simulink model "Controlled_simulink_model"  (R2021a)
settings: Solver=VariableStepAuto  StartTime=0  StopTime=150  FixedStep=0.001  MaxStep=1e-4  MinStep=1e-5  RelTol=1e-5
values from neighbouring files (symbols this model uses):
  Accel_bias = 0    [Controlled_model.m]
  Amps = C/1000    (= 0.7)    [Controlled_model.m]
  Ax = 0.0    (= 0)    [Controlled_model.m]
  Ay = 0.0    (= 0)    [Controlled_model.m]
  b = 1.144e-08    [Controlled_model.m]
  b_m = 2.415e-6    (= 2.415e-06)    [Controlled_model.m]
  CD = 60    [Controlled_model.m]
  d = 9.94e-10    [Controlled_model.m]
  g = 9.81    [Controlled_model.m]
  Gyro_bias = 0    [Controlled_model.m]
  Ixx = 7.5*10^(-3)    (= 0.0075)    [Controlled_model.m]
  Iyy = 7.5*10^(-3)    (= 0.0075)    [Controlled_model.m]
  Izz = 1.3*10^(-2)    (= 0.013)    [Controlled_model.m]
  Jr = 6.5*10^(-7)    (= 6.5e-07)    [Controlled_model.m]
  Kemf = 0.00255    [Controlled_model.m]
  Kt = Kemf    (= 0.00255)    [Controlled_model.m]
  l = 0.23    [Controlled_model.m]
  L = 0.001*R    (= 0.000117)    [Controlled_model.m]
  m = weight/g    (= 0.0289500509684)    [Controlled_model.m]
  PD = 120    [Controlled_model.m]
  R = 0.117    [Controlled_model.m]
undefined symbols (not defined in the file or in its folder): Ion, Lithium, sigbuilder_block
libraries: simulink x9, visionstatistics x1, spsControlledCurrentSourceLib x1, spsBatteryLib x1, spspowerguiLib x1
settings Model: Creator=Nicky  LastModifiedBy=YeBobo
settings SolverCC: MaxConsecutiveZCs=500  MaxConsecutiveMinStep=100  ZeroCrossAlgorithm=Adaptive  AlgebraicLoopSolver=LineSearch  AutoInsertRateTranBlk=on
settings DataIOCC: ReturnWorkspaceOutputs=off
settings DebuggingCC: MaxConsecutiveZCsMsg=none  SFMachineParentedDataDiag=warning  ArithmeticOperatorsInVariantConditions=warning
settings SFSimCC: SimUseLocalCustomCode=off  CustomCodeUndefinedFunction=UseInterfaceOnly
settings RTWCC: RTWUseLocalCustomCode=off
settings CodeAppCC: StateflowObjectComments=on
settings SimscapeCC: SimscapeNormalizeSystem=off

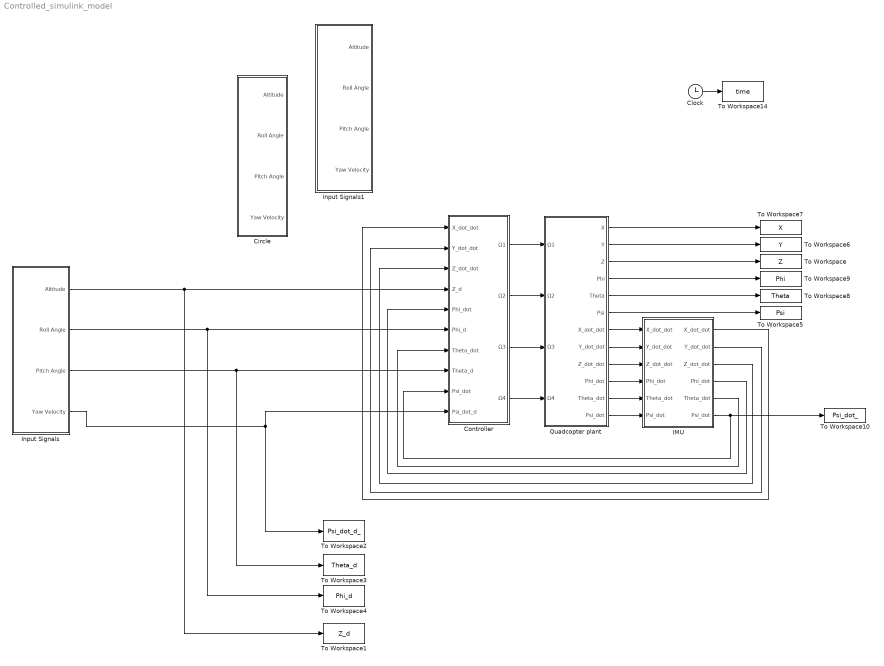
== system Controlled_simulink_model ==
  Circle : Subsystem  Tag=STV Subsys  LoadFcn=sigbuilder_block('load');  StartFcn=sigbuilder_block('start');  StopFcn=sigbuilder_block('stop');  ClipboardFcn=sigbuilder_block('clipboard');  mask(Sigbuilder block){tuvar=[0:10]}
      mask help: Simulink:masks:SigbuilderBlock_MD
      mask init:
      | if ~strcmp(get_param(bdroot(gcbh),'SimulationStatus'),'stopped') tuvar = sigbuilder_block('maskInit'); end
      settings: CopyFcn=sigbuilder_block('copy');  DeleteFcn=sigbuilder_block('delete');  ModelCloseFcn=sigbuilder_block('modelClose');  PreSaveFcn=sigbuilder_block('preSave');  PauseFcn=sigbuilder_block('pause');  ContinueFcn=sigbuilder_block('continue');  NameChangeFcn=sigbuilder_block('namechange');  OpenFcn=sigbuilder_block('open',[173.25 183.75 1012.5 456 ]);  CloseFcn=sigbuilder_block('close');
      mask Display: plot(0, 0, 100, 100,[2, 2, 32, 32, 2], [68, 8, 8, 68, 68],[32, 2], [38, 38], [32, 19, 2],[53, 60, 44], [32, 17, 17, 2],[16, 16, 31, 31]);txt = getActiveGroup(gcbh);text(2, 100, txt,'verticalAlignment', 'top');
  Clock : Clock
  Controller : Subsystem
  IMU : Subsystem
  Input Signals : Subsystem  Tag=STV Subsys  LoadFcn=sigbuilder_block('load');  StartFcn=sigbuilder_block('start');  StopFcn=sigbuilder_block('stop');  ClipboardFcn=sigbuilder_block('clipboard');  mask(Sigbuilder block){tuvar=[0:10]}
      mask help: Simulink:masks:SigbuilderBlock_MD
      mask init:
      | if ~strcmp(get_param(bdroot(gcbh),'SimulationStatus'),'stopped') tuvar = sigbuilder_block('maskInit'); end
      settings: CopyFcn=sigbuilder_block('copy');  DeleteFcn=sigbuilder_block('delete');  ModelCloseFcn=sigbuilder_block('modelClose');  PreSaveFcn=sigbuilder_block('preSave');  PauseFcn=sigbuilder_block('pause');  ContinueFcn=sigbuilder_block('continue');  NameChangeFcn=sigbuilder_block('namechange');  OpenFcn=sigbuilder_block('open',[133.8 179.4 1012.8 407.4 ]);  CloseFcn=sigbuilder_block('close');
      mask Display: plot(0, 0, 100, 100,[2, 2, 32, 32, 2], [68, 8, 8, 68, 68],[32, 2], [38, 38], [32, 19, 2],[53, 60, 44], [32, 17, 17, 2],[16, 16, 31, 31]);txt = getActiveGroup(gcbh);text(2, 100, txt,'verticalAlignment', 'top');
  Input Signals1 : Subsystem  Tag=STV Subsys  LoadFcn=sigbuilder_block('load');  StartFcn=sigbuilder_block('start');  StopFcn=sigbuilder_block('stop');  ClipboardFcn=sigbuilder_block('clipboard');  mask(Sigbuilder block){tuvar=[0:10]}
      mask help: Simulink:masks:SigbuilderBlock_MD
      mask init:
      | if ~strcmp(get_param(bdroot(gcbh),'SimulationStatus'),'stopped') tuvar = sigbuilder_block('maskInit'); end
      settings: CopyFcn=sigbuilder_block('copy');  DeleteFcn=sigbuilder_block('delete');  ModelCloseFcn=sigbuilder_block('modelClose');  PreSaveFcn=sigbuilder_block('preSave');  PauseFcn=sigbuilder_block('pause');  ContinueFcn=sigbuilder_block('continue');  NameChangeFcn=sigbuilder_block('namechange');  OpenFcn=sigbuilder_block('open',[369 232.5 1012.5 445.5 ]);  CloseFcn=sigbuilder_block('close');
      mask Display: plot(0, 0, 100, 100,[2, 2, 32, 32, 2], [68, 8, 8, 68, 68],[32, 2], [38, 38], [32, 19, 2],[53, 60, 44], [32, 17, 17, 2],[16, 16, 31, 31]);txt = getActiveGroup(gcbh);text(2, 100, txt,'verticalAlignment', 'top');
  Quadcopter plant : Subsystem
  To Workspace : ToWorkspace  VariableName=Z  SampleTime=0.001
      settings: Save2DSignal=2-D array (concatenate along first dimension)
  To Workspace1 : ToWorkspace  VariableName=Z_d  SampleTime=0.001
      settings: Save2DSignal=2-D array (concatenate along first dimension)
  To Workspace10 : ToWorkspace  VariableName=Psi_dot_  SampleTime=0.001
      settings: Save2DSignal=2-D array (concatenate along first dimension)
  To Workspace14 : ToWorkspace  VariableName=time  SampleTime=0.001
      settings: Save2DSignal=2-D array (concatenate along first dimension)
  To Workspace2 : ToWorkspace  VariableName=Psi_dot_d_  SampleTime=0.001
      settings: Save2DSignal=2-D array (concatenate along first dimension)
  To Workspace3 : ToWorkspace  VariableName=Theta_d  SampleTime=0.001
      settings: Save2DSignal=2-D array (concatenate along first dimension)
  To Workspace4 : ToWorkspace  VariableName=Phi_d  SampleTime=0.001
      settings: Save2DSignal=2-D array (concatenate along first dimension)
  To Workspace5 : ToWorkspace  VariableName=Psi  SampleTime=0.001
      settings: Save2DSignal=2-D array (concatenate along first dimension)
  To Workspace6 : ToWorkspace  VariableName=Y  SampleTime=0.001
      settings: Save2DSignal=2-D array (concatenate along first dimension)
  To Workspace7 : ToWorkspace  VariableName=X  SampleTime=0.001
      settings: Save2DSignal=2-D array (concatenate along first dimension)
  To Workspace8 : ToWorkspace  VariableName=Theta  SampleTime=0.001
      settings: Save2DSignal=2-D array (concatenate along first dimension)
  To Workspace9 : ToWorkspace  VariableName=Phi  SampleTime=0.001
      settings: Save2DSignal=2-D array (concatenate along first dimension)
  wires:
  Clock/1 -> To Workspace14/1
  Controller/1(Ω1) -> Quadcopter plant/1(Ω1)
  Controller/2(Ω2) -> Quadcopter plant/2(Ω2)
  Controller/3(Ω3) -> Quadcopter plant/3(Ω3)
  Controller/4(Ω4) -> Quadcopter plant/4(Ω4)
  IMU/6("Psi_dot ") -> Controller/9(Psi_dot), To Workspace10/1
  IMU/5("Theta_dot ") -> Controller/7(Theta_dot)
  IMU/3("Z_dot_dot ") -> Controller/3(Z_dot_dot)
  Quadcopter plant/1(X) -> To Workspace7/1
  Quadcopter plant/2(Y) -> To Workspace6/1
  Quadcopter plant/3(Z) -> To Workspace/1
  Quadcopter plant/7(X_dot_dot) -> IMU/1(X_dot_dot)
  Quadcopter plant/8("Y_dot_dot ") -> IMU/2(Y_dot_dot)
  Quadcopter plant/9(Z_dot_dot) -> IMU/3(Z_dot_dot)
  Quadcopter plant/11(Theta_dot) -> IMU/5(Theta_dot)
  Quadcopter plant/10(Phi_dot) -> IMU/4(Phi_dot)
  Quadcopter plant/12(Psi_dot) -> IMU/6(Psi_dot)
  Quadcopter plant/5(Theta) -> To Workspace8/1
  Quadcopter plant/6(Psi) -> To Workspace5/1
  IMU/2("Y_dot_dot ") -> Controller/2(Y_dot_dot)
  Input Signals/4(Yaw Velocity) -> Controller/10(Psi_dot_d), To Workspace2/1
  IMU/4("Phi_dot ") -> Controller/5(Phi_dot)
  Quadcopter plant/4(Phi) -> To Workspace9/1
  Input Signals/1(Altitude) -> To Workspace1/1, Controller/4(Z_d)
  Input Signals/2(Roll Angle) -> To Workspace4/1, Controller/6(Phi_d)
  Input Signals/3(Pitch Angle) -> To Workspace3/1, Controller/8(Theta_d)
  IMU/1("X_dot_dot ") -> Controller/1(X_dot_dot)

== system Controlled_simulink_model/Circle ==
  Demux : Demux  Tag=STV Demux
      settings: DisplayOption=none
  FromWs : FromWorkspace  Tag=STV FromWs  VariableName=tuvar
      SigBuilderData=|
      | common.afterFinalStr = 'Extrapolate'
      | common.sampleTime = 0
      | dataSet.timeRange = [0 150]
      | dataSet.name = 'Group 1'
      | sbobj.Groups.Name = 'Group 1'
      | sbobj.Groups.Signals(1).Name = 'Altitude'
      | sbobj.Groups.Signals(1).XData = [0 1 150]
      | sbobj.Groups.Signals(1).YData = [0 1 5]
      | sbobj.Groups.Signals(2).Name = 'Roll Angle'
      | sbobj.Groups.Signals(2).XData = [0 13 14 18 20 29 31 40 42 51 53 62 64 73 75 84 86 95 97 106 108 117 119 128 130 139 141 150]
      | sbobj.Groups.Signals(2).YData = [0 0 -0.1 -0.1 0.1 0.1 -0.1 -0.1 0.1 0.1 -0.1 -0.1 0.1 0.1 -0.1 -0.1 0.1 0.1 -0.1 -0.1 0.1 0.1 -0.1 -0.1 0.1 0.1 -0.1 -0.1]
      | sbobj.Groups.Signals(3).Name = 'Pitch Angle'
      | sbobj.Groups.Signals(3).XData = [0 7 8 12 14 23 25 34 36 45 47 56 58 67 69 78 80 89 91 100 102 111 113 122 124 133 135 144 146 150]
      | sbobj.Groups.Signals(3).YData = [0 0 -0.1 -0.1 0.1 0.1 -0.1 -0.1 0.1 0.1 -0.1 -0.1 0.1 0.1 -0.1 -0.1 0.1 0.1 -0.1 -0.1 0.1 0.1 -0.1 -0.1 0.1 0.1 -0.1 -0.1 0 0]
      | sbobj.Groups.Signals(4).Name = 'Yaw Velocity'
      | sbobj.Groups.Signals(4).XData = [0 150]
      | sbobj.Groups.Signals(4).YData = [0 0]
      | sbobj.Groups.TimeRange = [0 150]
  Altitude : Outport  Tag=STV Outport  VectorParamsAs1DForOutWhenUnconnected=off
  Roll Angle : Outport  Tag=STV Outport  Port=2  VectorParamsAs1DForOutWhenUnconnected=off
  Pitch Angle : Outport  Tag=STV Outport  Port=3  VectorParamsAs1DForOutWhenUnconnected=off
  Yaw Velocity : Outport  Tag=STV Outport  Port=4  VectorParamsAs1DForOutWhenUnconnected=off
  wires:
  FromWs/1 -> Demux/1
  Demux/1 -> Altitude/1
  Demux/2 -> Roll Angle/1
  Demux/3 -> Pitch Angle/1
  Demux/4 -> Yaw Velocity/1

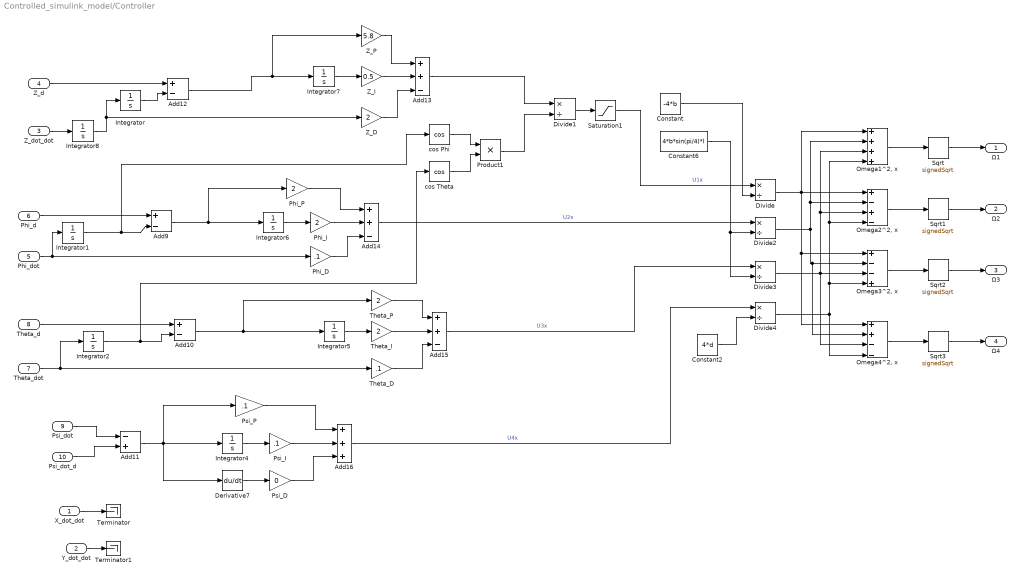
== system Controlled_simulink_model/Controller ==
  X_dot_dot : Inport
  Y_dot_dot : Inport  Port=2
  Z_dot_dot : Inport  Port=3
  Z_d : Inport  Port=4
  Phi_dot : Inport  Port=5
  Phi_d : Inport  Port=6
  Theta_dot : Inport  Port=7
  Theta_d : Inport  Port=8
  Psi_dot : Inport  Port=9
  Psi_dot_d : Inport  Port=10
  Add10 : Sum  Inputs=+-
  Add11 : Sum  Inputs=-+
  Add12 : Sum  Inputs=+-
  Add13 : Sum  Inputs=++-
  Add14 : Sum  Inputs=++-
  Add15 : Sum  Inputs=++-
  Add16 : Sum  Inputs=+++
  Add9 : Sum  Inputs=+-
  Constant : Constant  Value=-4*b
  Constant2 : Constant  Value=4*d
  Constant6 : Constant  Value=4*b*sin(pi/4)*l
  Derivative7 : Derivative
  Divide{,1..4} (5 alike) : Product  Inputs=*/
  Integrator : Integrator  LimitOutput=on  UpperSaturationLimit=0
  Integrator1 : Integrator  WrapState=on
  Integrator2 : Integrator  WrapState=on
  Integrator{4..8} (5 alike) : Integrator
  "Omega1^2, x" : Sum  Inputs=++++
  "Omega2^2, x" : Sum  Inputs=+-+-
  "Omega3^2, x" : Sum  Inputs=+--+
  "Omega4^2, x" : Sum  Inputs=++--
  Phi_D : Gain  Gain=.1
  Phi_I : Gain  Gain=2
  Phi_P : Gain  Gain=2
  Product1 : Product  RndMeth=Zero
  Psi_D : Gain  Gain=0
  Psi_I : Gain  Gain=.1
  Psi_P : Gain  Gain=.1
  Saturation1 : Saturate  UpperLimit=0  LowerLimit=-inf
  Sqrt{,1..3} (4 alike) : Sqrt  Operator=signedSqrt  SaturateOnIntegerOverflow=on
  Terminator : Terminator
  Terminator1 : Terminator
  Theta_D : Gain  Gain=.1
  Theta_I : Gain  Gain=2
  Theta_P : Gain  Gain=2
  Z_D : Gain  Gain=2
  "Z_I " : Gain  Gain=0.5
  Z_P : Gain  Gain=5.8
  cos Phi : Trigonometry  Operator=cos
  cos Theta : Trigonometry  Operator=cos
  Ω1 : Outport  VectorParamsAs1DForOutWhenUnconnected=off
  Ω2 : Outport  Port=2  VectorParamsAs1DForOutWhenUnconnected=off
  Ω3 : Outport  Port=3  VectorParamsAs1DForOutWhenUnconnected=off
  Ω4 : Outport  Port=4  VectorParamsAs1DForOutWhenUnconnected=off
  wires:
  Z_D/1 -> Add13/3
  Theta_I/1 -> Add15/2
  Add12/1 -> Z_P/1, Integrator7/1
  Z_dot_dot/1 -> Integrator8/1
  Add11/1 -> Derivative7/1, Integrator4/1, Psi_P/1
  "Z_I "/1 -> Add13/2
  Theta_P/1 -> Add15/1
  Integrator4/1 -> Psi_I/1
  Integrator7/1 -> "Z_I "/1
  Add9/1 -> Integrator6/1, Phi_P/1
  Derivative7/1 -> Psi_D/1
  Psi_D/1 -> Add16/3
  Psi_I/1 -> Add16/2
  Integrator6/1 -> Phi_I/1
  cos Theta/1 -> Product1/2
  Add13/1 -> Divide1/1
  Phi_dot/1 -> Phi_D/1, Integrator1/1
  Phi_D/1 -> Add14/3
  cos Phi/1 -> Product1/1
  Divide1/1 -> Saturation1/1
  Theta_D/1 -> Add15/3
  Integrator5/1 -> Theta_I/1
  Add10/1 -> Theta_P/1, Integrator5/1
  Product1/1 -> Divide1/2
  Phi_I/1 -> Add14/2
  Theta_dot/1 -> Integrator2/1, Theta_D/1
  Phi_P/1 -> Add14/1
  Psi_P/1 -> Add16/1
  Z_P/1 -> Add13/1
  Constant6/1 -> Divide3/2, Divide2/2
  Add14/1 -> Divide2/1  "U2x"
  Add15/1 -> Divide3/1  "U3x"
  Saturation1/1 -> Divide/1  "U1x"
  Constant/1 -> Divide/2
  Constant2/1 -> Divide4/2
  Add16/1 -> Divide4/1  "U4x"
  Sqrt/1 -> Ω1/1
  Sqrt1/1 -> Ω2/1
  Sqrt2/1 -> Ω3/1
  Sqrt3/1 -> Ω4/1
  Divide4/1 -> "Omega3^2, x"/4, "Omega2^2, x"/4, "Omega1^2, x"/4, "Omega4^2, x"/4
  Divide2/1 -> "Omega4^2, x"/2, "Omega3^2, x"/2, "Omega2^2, x"/2, "Omega1^2, x"/2
  Divide3/1 -> "Omega4^2, x"/3, "Omega3^2, x"/3, "Omega2^2, x"/3, "Omega1^2, x"/3
  Divide/1 -> "Omega4^2, x"/1, "Omega3^2, x"/1, "Omega2^2, x"/1, "Omega1^2, x"/1
  "Omega1^2, x"/1 -> Sqrt/1
  "Omega2^2, x"/1 -> Sqrt1/1
  "Omega3^2, x"/1 -> Sqrt2/1
  "Omega4^2, x"/1 -> Sqrt3/1
  Z_d/1 -> Add12/1
  Phi_d/1 -> Add9/1
  Integrator1/1 -> cos Phi/1, Add9/2
  Integrator2/1 -> cos Theta/1, Add10/2
  Theta_d/1 -> Add10/1
  Psi_dot/1 -> Add11/1
  Psi_dot_d/1 -> Add11/2
  Integrator/1 -> Add12/2
  Integrator8/1 -> Z_D/1, Integrator/1
  X_dot_dot/1 -> Terminator/1
  Y_dot_dot/1 -> Terminator1/1

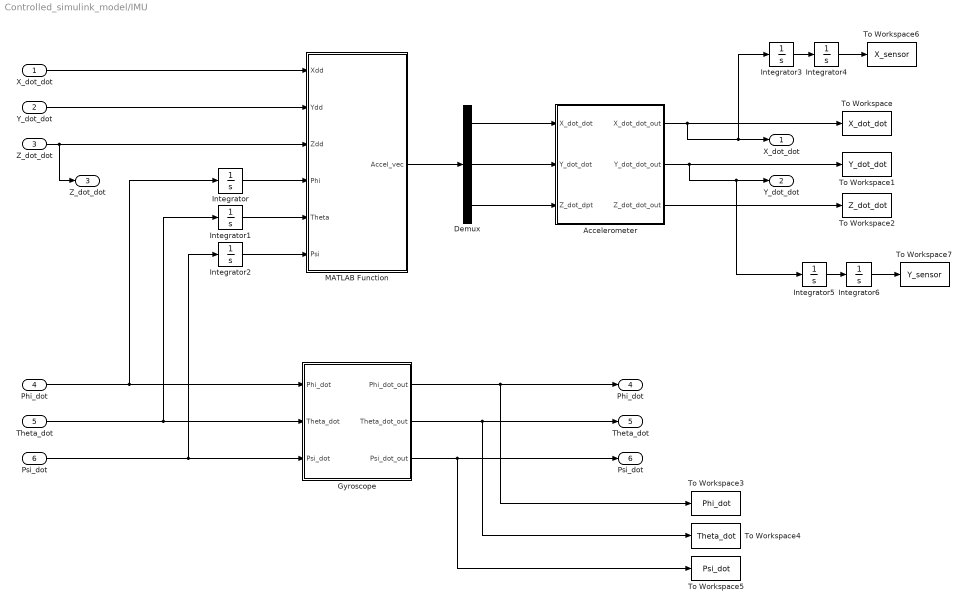
== system Controlled_simulink_model/IMU ==
  X_dot_dot : Inport
  Y_dot_dot : Inport  Port=2
  Z_dot_dot : Inport  Port=3
  Phi_dot : Inport  Port=4
  Theta_dot : Inport  Port=5
  Psi_dot : Inport  Port=6
  Accelerometer : Subsystem
  Demux : Demux  Outputs=3
  Gyroscope : Subsystem
  Integrator : Integrator  WrapState=on
  Integrator1 : Integrator  WrapState=on
  Integrator{2..6} (5 alike) : Integrator
  MATLAB Function : MATLAB Function  TreatAsAtomicUnit=on
  To Workspace : ToWorkspace  VariableName=X_dot_dot  SampleTime=0.001
      settings: Save2DSignal=2-D array (concatenate along first dimension)
  To Workspace1 : ToWorkspace  VariableName=Y_dot_dot  SampleTime=0.001
      settings: Save2DSignal=2-D array (concatenate along first dimension)
  To Workspace2 : ToWorkspace  VariableName=Z_dot_dot  SampleTime=0.001
      settings: Save2DSignal=2-D array (concatenate along first dimension)
  To Workspace3 : ToWorkspace  VariableName=Phi_dot  SampleTime=0.001
      settings: Save2DSignal=2-D array (concatenate along first dimension)
  To Workspace4 : ToWorkspace  VariableName=Theta_dot  SampleTime=0.001
      settings: Save2DSignal=2-D array (concatenate along first dimension)
  To Workspace5 : ToWorkspace  VariableName=Psi_dot  SampleTime=0.001
      settings: Save2DSignal=2-D array (concatenate along first dimension)
  To Workspace6 : ToWorkspace  VariableName=X_sensor  SampleTime=0.001
      settings: Save2DSignal=2-D array (concatenate along first dimension)
  To Workspace7 : ToWorkspace  VariableName=Y_sensor  SampleTime=0.001
      settings: Save2DSignal=2-D array (concatenate along first dimension)
  "X_dot_dot " : Outport  VectorParamsAs1DForOutWhenUnconnected=off
  "Y_dot_dot " : Outport  Port=2  VectorParamsAs1DForOutWhenUnconnected=off
  "Z_dot_dot " : Outport  Port=3  VectorParamsAs1DForOutWhenUnconnected=off
  "Phi_dot " : Outport  Port=4  VectorParamsAs1DForOutWhenUnconnected=off
  "Theta_dot " : Outport  Port=5  VectorParamsAs1DForOutWhenUnconnected=off
  "Psi_dot " : Outport  Port=6  VectorParamsAs1DForOutWhenUnconnected=off
  wires:
  Phi_dot/1 -> Integrator/1, Gyroscope/1(Phi_dot)
  Theta_dot/1 -> Integrator1/1, Gyroscope/2(Theta_dot)
  Psi_dot/1 -> Integrator2/1, Gyroscope/3(Psi_dot)
  Gyroscope/2(Theta_dot_out) -> "Theta_dot "/1, To Workspace4/1
  Gyroscope/1(Phi_dot_out) -> "Phi_dot "/1, To Workspace3/1
  Accelerometer/1(X_dot_dot_out) -> To Workspace/1, Integrator3/1, "X_dot_dot "/1
  Accelerometer/3(Z_dot_dot_out) -> To Workspace2/1
  Gyroscope/3(Psi_dot_out) -> "Psi_dot "/1, To Workspace5/1
  X_dot_dot/1 -> MATLAB Function/1(Xdd)
  Y_dot_dot/1 -> MATLAB Function/2(Ydd)
  Z_dot_dot/1 -> "Z_dot_dot "/1, MATLAB Function/3(Zdd)
  Integrator/1 -> MATLAB Function/4(Phi)
  Integrator2/1 -> MATLAB Function/6(Psi)
  Integrator1/1 -> MATLAB Function/5(Theta)
  MATLAB Function/1(Accel_vec) -> Demux/1
  Demux/2 -> Accelerometer/2("Y_dot_dot ")
  Demux/1 -> Accelerometer/1(X_dot_dot)
  Demux/3 -> Accelerometer/3("Z_dot_dpt ")
  Integrator3/1 -> Integrator4/1
  Integrator4/1 -> To Workspace6/1
  Integrator6/1 -> To Workspace7/1
  Accelerometer/2(Y_dot_dot_out) -> Integrator5/1, "Y_dot_dot "/1, To Workspace1/1
  Integrator5/1 -> Integrator6/1

== system Controlled_simulink_model/Input Signals ==
  Demux : Demux  Tag=STV Demux
      settings: DisplayOption=none
  FromWs : FromWorkspace  Tag=STV FromWs  VariableName=tuvar
      SigBuilderData=|
      | common.afterFinalStr = 'Extrapolate'
      | common.sampleTime = 0
      | dataSet.timeRange = [0 150]
      | dataSet.name = 'Group 1'
      | sbobj.Groups.Name = 'Group 1'
      | sbobj.Groups.Signals(1).Name = 'Altitude'
      | sbobj.Groups.Signals(1).XData = [0 60 60 150]
      | sbobj.Groups.Signals(1).YData = [-1 -1 -2 -2]
      | sbobj.Groups.Signals(2).Name = 'Roll Angle'
      | sbobj.Groups.Signals(2).XData = [0 2 3 5 6 8 9 11 12 30 31 33 34 36 37 39 40 75 76 78 79 81 82 84 85 103 104 106 107 109 110 112 113 150]
      | sbobj.Groups.Signals(2).YData = [0 0 0.2 0.2 0 0 -0.2 -0.2 0 0 -0.2 -0.2 0 0 0.2 0.2 0 0 0.2 0.2 0 0 -0.2 -0.2 0 0 -0.2 -0.2 0 0 0.2 0.2 0 0]
      | sbobj.Groups.Signals(3).Name = 'Pitch Angle'
      | sbobj.Groups.Signals(3).XData = [0 16 17 19 20 22 23 25 26 44 45 47 48 50 51 53 54 89 90 92 93 95 96 98 99 117 117 118 120 121 123 124 126 127 140.4 150]
      | sbobj.Groups.Signals(3).YData = [0 0 0.2 0.2 0 0 -0.2 -0.2 0 0 -0.2 -0.2 0 0 0.2 0.2 0 0 0.2 0.2 0 0 -0.2 -0.2 0 0 0.005 -0.2 -0.2 0 0 0.2 0.2 0 0 0]
      | sbobj.Groups.Signals(4).Name = 'Yaw Velocity'
      | sbobj.Groups.Signals(4).XData = [0 65 66 70 71 150]
      | sbobj.Groups.Signals(4).YData = [0 0 0.5 0.5 0 0]
      | sbobj.Groups.TimeRange = [0 150]
  Altitude : Outport  Tag=STV Outport  VectorParamsAs1DForOutWhenUnconnected=off
  Roll Angle : Outport  Tag=STV Outport  Port=2  VectorParamsAs1DForOutWhenUnconnected=off
  Pitch Angle : Outport  Tag=STV Outport  Port=3  VectorParamsAs1DForOutWhenUnconnected=off
  Yaw Velocity : Outport  Tag=STV Outport  Port=4  VectorParamsAs1DForOutWhenUnconnected=off
  wires:
  FromWs/1 -> Demux/1
  Demux/1 -> Altitude/1
  Demux/2 -> Roll Angle/1
  Demux/3 -> Pitch Angle/1
  Demux/4 -> Yaw Velocity/1

== system Controlled_simulink_model/Input Signals1 ==
  Demux : Demux  Tag=STV Demux
      settings: DisplayOption=none
  FromWs : FromWorkspace  Tag=STV FromWs  VariableName=tuvar
      SigBuilderData=|
      | common.afterFinalStr = 'Extrapolate'
      | common.sampleTime = 0
      | dataSet.timeRange = [0 150]
      | dataSet.name = 'Group 1'
      | sbobj.Groups.Name = 'Group 1'
      | sbobj.Groups.Signals(1).Name = 'Altitude'
      | sbobj.Groups.Signals(1).XData = [0 150]
      | sbobj.Groups.Signals(1).YData = [-1 -10]
      | sbobj.Groups.Signals(2).Name = 'Roll Angle'
      | sbobj.Groups.Signals(2).XData = [0 2 3 5 6 16 17 19 20 30 31 33 34 44 45 47 48 103 104 106 107 109 110 112 113 150]
      | sbobj.Groups.Signals(2).YData = [0 0 0.2 0.2 0 0 -0.2 -0.2 0 0 0.2 0.2 0 0 -0.2 -0.2 0 0 -0.2 -0.2 0 0 0.2 0.2 0 0]
      | sbobj.Groups.Signals(3).Name = 'Pitch Angle'
      | sbobj.Groups.Signals(3).XData = [0 140.4 150]
      | sbobj.Groups.Signals(3).YData = [0 0 0]
      | sbobj.Groups.Signals(4).Name = 'Yaw Velocity'
      | sbobj.Groups.Signals(4).XData = [0 65 66 70 71 150]
      | sbobj.Groups.Signals(4).YData = [0 0 0.5 0.5 0 0]
      | sbobj.Groups.TimeRange = [0 150]
  Altitude : Outport  Tag=STV Outport  VectorParamsAs1DForOutWhenUnconnected=off
  Roll Angle : Outport  Tag=STV Outport  Port=2  VectorParamsAs1DForOutWhenUnconnected=off
  Pitch Angle : Outport  Tag=STV Outport  Port=3  VectorParamsAs1DForOutWhenUnconnected=off
  Yaw Velocity : Outport  Tag=STV Outport  Port=4  VectorParamsAs1DForOutWhenUnconnected=off
  wires:
  FromWs/1 -> Demux/1
  Demux/1 -> Altitude/1
  Demux/2 -> Roll Angle/1
  Demux/3 -> Pitch Angle/1
  Demux/4 -> Yaw Velocity/1

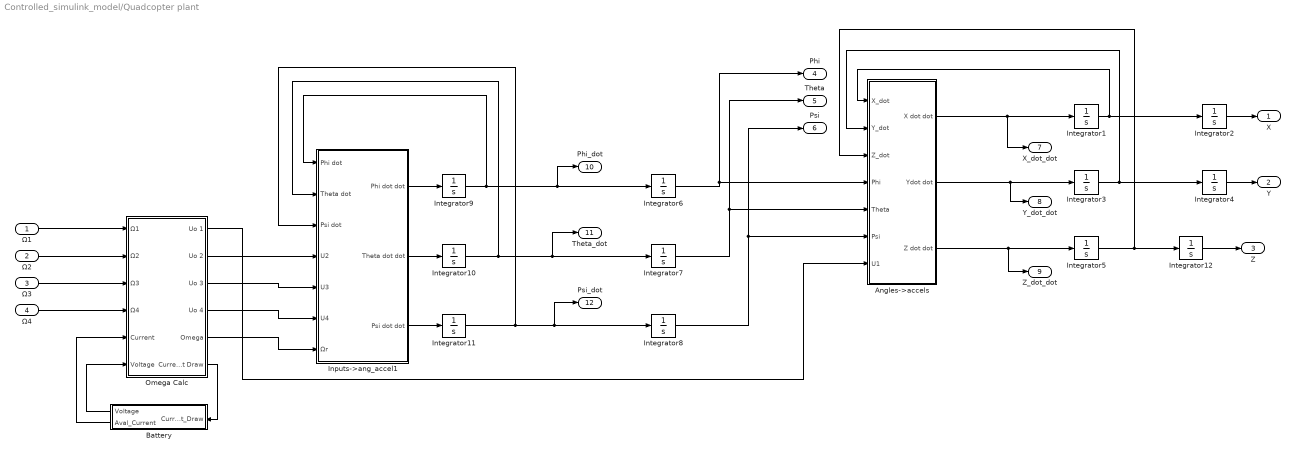
== system Controlled_simulink_model/Quadcopter plant ==
  Ω1 : Inport
  Ω2 : Inport  Port=2
  Ω3 : Inport  Port=3
  Ω4 : Inport  Port=4
  Angles->accels : Subsystem
  Battery : Subsystem
  Inputs->ang_accel1 : Subsystem
  Integrator{1..5,8..9} (7 alike) : Integrator
  Integrator10 : Integrator  IgnoreLimit=on
  Integrator11 : Integrator  UpperSaturationLimit=10000  LowerSaturationLimit=-10000
  Integrator12 : Integrator  LimitOutput=on  UpperSaturationLimit=0
  Integrator6 : Integrator  WrapState=on
  Integrator7 : Integrator  WrapState=on
  Omega Calc : Subsystem
  X : Outport  VectorParamsAs1DForOutWhenUnconnected=off
  Y : Outport  Port=2  VectorParamsAs1DForOutWhenUnconnected=off
  Z : Outport  Port=3  VectorParamsAs1DForOutWhenUnconnected=off
  Phi : Outport  Port=4  VectorParamsAs1DForOutWhenUnconnected=off
  Theta : Outport  Port=5  VectorParamsAs1DForOutWhenUnconnected=off
  Psi : Outport  Port=6  VectorParamsAs1DForOutWhenUnconnected=off
  X_dot_dot : Outport  Port=7  VectorParamsAs1DForOutWhenUnconnected=off
  "Y_dot_dot " : Outport  Port=8  VectorParamsAs1DForOutWhenUnconnected=off
  Z_dot_dot : Outport  Port=9  VectorParamsAs1DForOutWhenUnconnected=off
  Phi_dot : Outport  Port=10  VectorParamsAs1DForOutWhenUnconnected=off
  Theta_dot : Outport  Port=11  VectorParamsAs1DForOutWhenUnconnected=off
  Psi_dot : Outport  Port=12  VectorParamsAs1DForOutWhenUnconnected=off
  wires:
  Integrator7/1 -> Angles->accels/5(Theta), Theta/1
  Integrator6/1 -> Angles->accels/4(Phi), Phi/1
  Inputs->ang_accel1/2(Theta dot dot) -> Integrator10/1
  Inputs->ang_accel1/1(Phi dot dot) -> Integrator9/1
  Inputs->ang_accel1/3(Psi dot dot) -> Integrator11/1
  Omega Calc/5(Omega) -> Inputs->ang_accel1/7(Ωr)
  Omega Calc/4(Uo 4) -> Inputs->ang_accel1/6(U4)
  Omega Calc/3(Uo 3) -> Inputs->ang_accel1/5(U3)
  Omega Calc/2(Uo 2) -> Inputs->ang_accel1/4(U2)
  Omega Calc/1(Uo 1) -> Angles->accels/7(U1)
  Ω1/1 -> Omega Calc/1(Ω1)
  Ω2/1 -> Omega Calc/2(Ω2)
  Ω3/1 -> Omega Calc/3(Ω3)
  Ω4/1 -> Omega Calc/4(Ω4)
  Integrator9/1 -> Inputs->ang_accel1/1(Phi dot), Phi_dot/1, Integrator6/1
  Integrator11/1 -> Inputs->ang_accel1/3(Psi dot), Integrator8/1, Psi_dot/1
  Integrator10/1 -> Inputs->ang_accel1/2(Theta dot), Integrator7/1, Theta_dot/1
  Angles->accels/1(X dot dot) -> X_dot_dot/1, Integrator1/1
  Omega Calc/6(Current Draw) -> Battery/1(Current_Draw)
  Battery/1(Voltage) -> Omega Calc/6(Voltage)
  Battery/2(Aval_Current) -> Omega Calc/5(Current)
  Integrator1/1 -> Angles->accels/1(X_dot), Integrator2/1
  Integrator2/1 -> X/1
  Integrator3/1 -> Angles->accels/2(Y_dot), Integrator4/1
  Angles->accels/2(Ydot dot) -> "Y_dot_dot "/1, Integrator3/1
  Integrator4/1 -> Y/1
  Integrator5/1 -> Angles->accels/3(Z_dot), Integrator12/1
  Angles->accels/3(Z dot dot) -> Integrator5/1, Z_dot_dot/1
  Integrator12/1 -> Z/1
  Integrator8/1 -> Angles->accels/6(Psi), Psi/1

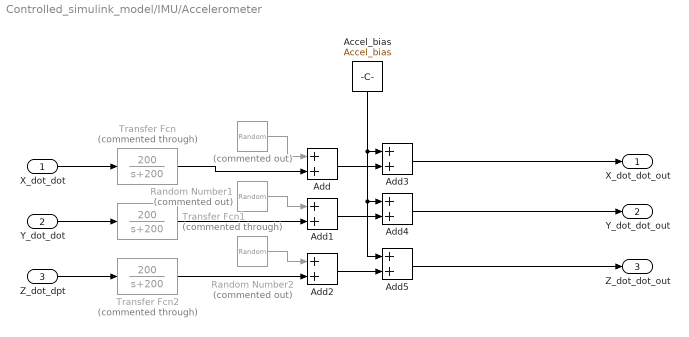
== system Controlled_simulink_model/IMU/Accelerometer ==
  X_dot_dot : Inport
  "Y_dot_dot " : Inport  Port=2
  "Z_dot_dpt " : Inport  Port=3
  " " : RandomNumber  Commented=on  Variance=0.0001  Seed=1  SampleTime=0.001
  Accel_bias : Constant  Value=Accel_bias
  Add{,1..5} (6 alike) : Sum
  Random Number1 : RandomNumber  Commented=on  Variance=0.0001  Seed=2  SampleTime=0.001
  Random Number2 : RandomNumber  Commented=on  Mean=0.000  Variance=0.0001  Seed=3  SampleTime=0.001
  Transfer Fcn : TransferFcn  Commented=through  Numerator=[200]  Denominator=[1 200]
  Transfer Fcn1 : TransferFcn  Commented=through  Numerator=[200]  Denominator=[1 200]
  Transfer Fcn2 : TransferFcn  Commented=through  Numerator=[200]  Denominator=[1 200]
  X_dot_dot_out : Outport  VectorParamsAs1DForOutWhenUnconnected=off
  Y_dot_dot_out : Outport  Port=2  VectorParamsAs1DForOutWhenUnconnected=off
  Z_dot_dot_out : Outport  Port=3  VectorParamsAs1DForOutWhenUnconnected=off
  wires:
  X_dot_dot/1 -> Transfer Fcn/1
  "Y_dot_dot "/1 -> Transfer Fcn1/1
  Accel_bias/1 -> Add5/1, Add4/1, Add3/1
  Add/1 -> Add3/2
  Add2/1 -> Add5/2
  Add1/1 -> Add4/2
  " "/1 -> Add/1
  Random Number1/1 -> Add1/1
  Random Number2/1 -> Add2/1
  "Z_dot_dpt "/1 -> Transfer Fcn2/1
  Add3/1 -> X_dot_dot_out/1
  Add4/1 -> Y_dot_dot_out/1
  Add5/1 -> Z_dot_dot_out/1
  Transfer Fcn/1 -> Add/2
  Transfer Fcn1/1 -> Add1/2
  Transfer Fcn2/1 -> Add2/2

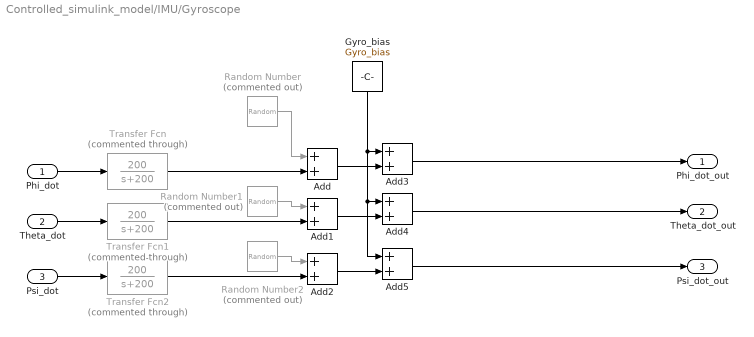
== system Controlled_simulink_model/IMU/Gyroscope ==
  Phi_dot : Inport
  Theta_dot : Inport  Port=2
  Psi_dot : Inport  Port=3
  Add{,1..5} (6 alike) : Sum
  Gyro_bias : Constant  Value=Gyro_bias
  Random Number : RandomNumber  Commented=on  Variance=0.0001  Seed=4  SampleTime=0.001
  Random Number1 : RandomNumber  Commented=on  Variance=0.0001  Seed=5  SampleTime=0.001
  Random Number2 : RandomNumber  Commented=on  Variance=0.0001  Seed=6  SampleTime=0.001
  Transfer Fcn : TransferFcn  Commented=through  Numerator=[200]  Denominator=[1 200]
  Transfer Fcn1 : TransferFcn  Commented=through  Numerator=[200]  Denominator=[1 200]
  Transfer Fcn2 : TransferFcn  Commented=through  Numerator=[200]  Denominator=[1 200]
  Phi_dot_out : Outport  VectorParamsAs1DForOutWhenUnconnected=off
  Theta_dot_out : Outport  Port=2  VectorParamsAs1DForOutWhenUnconnected=off
  Psi_dot_out : Outport  Port=3  VectorParamsAs1DForOutWhenUnconnected=off
  wires:
  Phi_dot/1 -> Transfer Fcn/1
  Theta_dot/1 -> Transfer Fcn1/1
  Psi_dot/1 -> Transfer Fcn2/1
  Add/1 -> Add3/2
  Add1/1 -> Add4/2
  Add2/1 -> Add5/2
  Gyro_bias/1 -> Add5/1, Add4/1, Add3/1
  Random Number/1 -> Add/1
  Random Number1/1 -> Add1/1
  Random Number2/1 -> Add2/1
  Add3/1 -> Phi_dot_out/1
  Add4/1 -> Theta_dot_out/1
  Add5/1 -> Psi_dot_out/1
  Transfer Fcn2/1 -> Add2/2
  Transfer Fcn1/1 -> Add1/2
  Transfer Fcn/1 -> Add/2

== system Controlled_simulink_model/Quadcopter plant/Angles->accels ==
  X_dot : Inport
  Y_dot : Inport  Port=2
  Z_dot : Inport  Port=3
  Phi : Inport  Port=4
  Theta : Inport  Port=5
  Psi : Inport  Port=6
  U1 : Inport  Port=7
  Constant : Constant  Value=m
  Divide : Product  Inputs=*/
  Subsystem : Subsystem
  Subsystem1 : Subsystem
  Subsystem2 : Subsystem
  X dot dot : Outport  VectorParamsAs1DForOutWhenUnconnected=off
  Ydot dot : Outport  Port=2  VectorParamsAs1DForOutWhenUnconnected=off
  Z dot dot : Outport  Port=3  VectorParamsAs1DForOutWhenUnconnected=off
  wires:
  Phi/1 -> Subsystem2/2(Phi), Subsystem1/2(Phi), Subsystem/2(Phi)
  U1/1 -> Divide/1
  Constant/1 -> Divide/2
  Divide/1 -> Subsystem/5(U1/M), Subsystem2/4(U1/m), Subsystem1/5(U1/M)
  Subsystem/1(X_dot_dot) -> X dot dot/1
  Subsystem1/1(Y_dot_dot) -> Ydot dot/1
  Subsystem2/1(Z_dot_dot) -> Z dot dot/1
  Theta/1 -> Subsystem2/3(Theta), Subsystem1/3(Theta), Subsystem/3(Theta)
  Psi/1 -> Subsystem1/4(Psi), Subsystem/4(Psi)
  X_dot/1 -> Subsystem/1(X_dot)
  Y_dot/1 -> Subsystem1/1(Y_dot)
  Z_dot/1 -> Subsystem2/1(Z_dot)

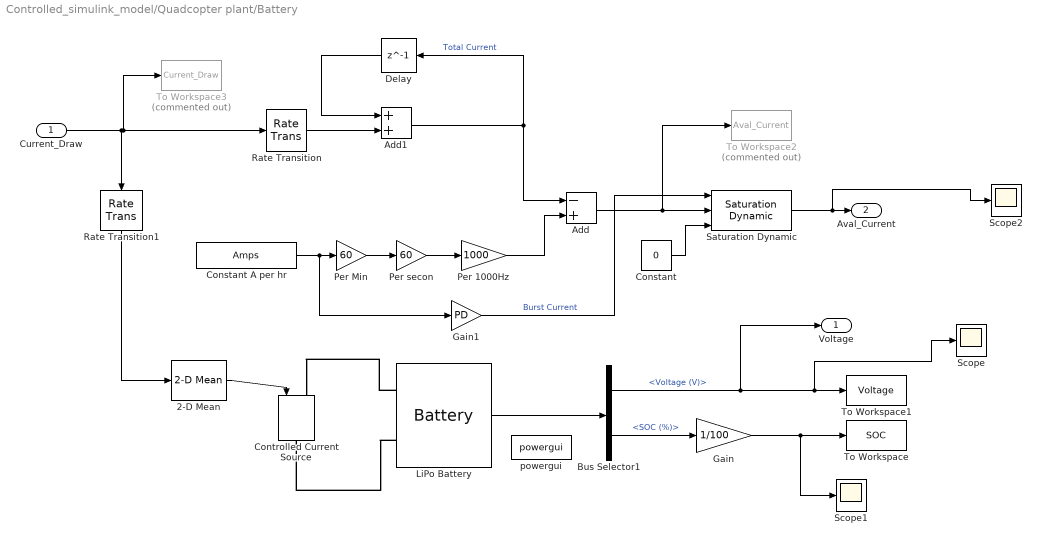
== system Controlled_simulink_model/Quadcopter plant/Battery ==
  Current_Draw : Inport
  2-D Mean : visionstatistics/2-D Mean  run=on  reset_popup=None  directionMode=Entire input  dimension=1  treatSBRowAsCol=on  outputLastDataTypeStr=Inherit: Same as accumulator  accumMode=Binary point scaling  accumWordLength=32  accumFracLength=0  accumLastDataTypeStr=fixdt([],32,0)  roiEnable=off  roiType=Rectangles  roiPortion=Entire ROI  roiOutput=Individual statistics for each ROI  roiFlag=off  roundingMode=Floor  overflowMode=off  accumDataTypeStr=fixdt([],32,0)  outputDataTypeStr=Inherit: Same as accumulator  outputMin=[]  outputMax=[]
      settings: SourceProductBaseCode=VP
  Add : Sum  Inputs=-+
  Add1 : Sum
  Bus Selector1 : BusSelector  OutputSignals=Voltage (V),SOC (%)
  Constant : Constant  Value=0
  Constant A per hr : Constant  Value=Amps
  Controlled Current Source : spsControlledCurrentSourceLib/Controlled Current Source  Initialize=on  Source_Type=DC  Amplitude=0  Phase=0  Frequency=0  Measurements=None
  Delay : Delay  DelayLength=1  InitialCondition=0
  Gain : Gain  Gain=1/100
  Gain1 : Gain  Gain=PD
  "LiPo Battery " : spsBatteryLib/Battery  BatType=Lithium-Ion  ShowTempParam=off  ThermalPreset=no  ShowAgeParam=off  NomV=11.1  NomQ=.7  SOC=100  Batt_Tr=1  PresetModel=off  MaxQ=0.7  MinV=8.325  FullV=11.7  Dis_rate=.7  R=.11  Normal_OP=.7  expZone="[11.7   0.5]"  current=CD*Amps  Units=Ampere-hour  Tci=20  NomT=25  T2=0  MaxQ2=2.208  FullV2=3.45  Normal_OP2=2.8  expZone2="[3.22        0.23]"  Rca=0.6  ti=1000  Dp=0  Neq0=0  Tsim=1e6  Ta1=25  Qeol=5.4*0.9  Reol=0.013333*1.2  Char_age=[2.3478, 3]  Dis_age=[2.3478, 10]  N1=1500  N2=10500  N3=1000  N4=1400  Ta2=45  N5=950
  Per 1000Hz : Gain  Gain=1000
  Per Min : Gain  Gain=60
  Per secon : Gain  Gain=60
  Rate Transition : RateTransition  OutPortSampleTimeMultiple=0  OutPortSampleTime=0.001
  Rate Transition1 : RateTransition  OutPortSampleTimeMultiple=0  OutPortSampleTime=0.001
  Saturation Dynamic : simulink/Discontinuities/Saturation Dynamic  OutMin=[]  OutMax=[]  OutDataTypeStr=Inherit: Same as second input  OutDataType=fixdt(1, 16)  OutScaling=2^-10  DoSatur=on
  Scope : Scope
  Scope1 : Scope
  Scope2 : Scope
  To Workspace : ToWorkspace  VariableName=SOC  SampleTime=0.001
      settings: Save2DSignal=2-D array (concatenate along first dimension)
  To Workspace1 : ToWorkspace  VariableName=Voltage  SampleTime=0.001
      settings: Save2DSignal=2-D array (concatenate along first dimension)
  To Workspace2 : ToWorkspace  Commented=on  VariableName=Aval_Current  SampleTime=.1
      settings: Save2DSignal=2-D array (concatenate along first dimension)
  To Workspace3 : ToWorkspace  Commented=on  VariableName=Current_Draw  SampleTime=.1
      settings: Save2DSignal=2-D array (concatenate along first dimension)
  powergui : spspowerguiLib/powergui  SimulationMode=Continuous  SampleTime=0.001  frequency=60  Iterations=50  frequencyindice=0  Pbase=100e6  ErrMax=1e-4  UnitsV=kV  UnitsW=MW  buscounter=0  FunctionMessages=off  echomessages=off  EnableUseOfTLC=off  CurrentSourceSwitches=off  DisableSnubberDevices=off  DisableRonSwitches=off  DisableVfSwitches=off  DisplayEquations=off  AutomaticDiscreteSolvers=off  SolverType=Tustin/Backward Euler (TBE)  Interpol=off  ExternalGateDelay=off  methode=off  Ts=100  x0status=blocks  SPID=on  SwTol=0  HookPort=off  NonlinearTolerance=1e-4  nMaxIteration=100  ContinueOnMaxIteration=off  RestoreLinks=warning  ResistiveCurrentMeasurement=off  Frange=[0:2:500]  Ylog=off  Xlog=on  ShowGrid=off  save=off  variable=ZData  structure=0  ZoomFFT=on  StartTime=0.0  cycles=1  DisplayStyle=1  fundamental=60  FreqAxis=off  MaxFrequency=1000  frequencyindicesteady=1  RmsSteady=1  display=off
  Voltage : Outport  VectorParamsAs1DForOutWhenUnconnected=off
  Aval_Current : Outport  Port=2  VectorParamsAs1DForOutWhenUnconnected=off
  wires:
  Per Min/1 -> Per secon/1
  Constant A per hr/1 -> Gain1/1, Per Min/1
  Per secon/1 -> Per 1000Hz/1
  Per 1000Hz/1 -> Add/2
  Add1/1 -> Add/1, Delay/1  "Total Current"
  Rate Transition/1 -> Add1/2
  Delay/1 -> Add1/1
  Constant/1 -> Saturation Dynamic/3
  Current_Draw/1 -> To Workspace3/1, Rate Transition/1, Rate Transition1/1
  Bus Selector1/1 -> Voltage/1, Scope/1, To Workspace1/1  "<Voltage (V)>"
  Bus Selector1/2 -> Gain/1  "<SOC (%)>"
  "LiPo Battery "/1 -> Bus Selector1/1
  Add/1 -> To Workspace2/1, Saturation Dynamic/2
  Saturation Dynamic/1 -> Scope2/1, Aval_Current/1
  Gain1/1 -> Saturation Dynamic/1  "Burst Current"
  Gain/1 -> Scope1/1, To Workspace/1
  Rate Transition1/1 -> 2-D Mean/1
  2-D Mean/1 -> Controlled Current Source/1
  connections:
  "LiPo Battery "/LConn1 -- Controlled Current Source/LConn1
  "LiPo Battery "/LConn2 -- Controlled Current Source/RConn1

== system Controlled_simulink_model/Quadcopter plant/Inputs->ang_accel1 ==
  Phi dot : Inport
  Theta dot : Inport  Port=2
  Psi dot : Inport  Port=3
  U2 : Inport  Port=4
  U3 : Inport  Port=5
  U4 : Inport  Port=6
  Ωr : Inport  Port=7
  Subsystem : Subsystem
  Subsystem1 : Subsystem
  Subsystem2 : Subsystem
  Phi dot dot : Outport  VectorParamsAs1DForOutWhenUnconnected=off
  Theta dot dot : Outport  Port=2  VectorParamsAs1DForOutWhenUnconnected=off
  Psi dot dot : Outport  Port=3  VectorParamsAs1DForOutWhenUnconnected=off
  wires:
  U3/1 -> Subsystem2/3(U3)
  U4/1 -> Subsystem1/3(U4)
  Subsystem/1(Phi_dot_dot) -> Phi dot dot/1
  U2/1 -> Subsystem/1(U2)
  Ωr/1 -> Subsystem/4(Ωr), Subsystem2/1(Ωr)
  Psi dot/1 -> Subsystem2/2(Psi_dot), Subsystem/3(Psi_dot)
  Subsystem2/1(Theta_dot_dot) -> Theta dot dot/1
  Subsystem1/1(Psi_dot_dot) -> Psi dot dot/1
  Theta dot/1 -> Subsystem/2(Theta_dot), Subsystem1/2(Theta_dot)
  Phi dot/1 -> Subsystem2/4(Phi_dot), Subsystem1/1(Phi_dot)

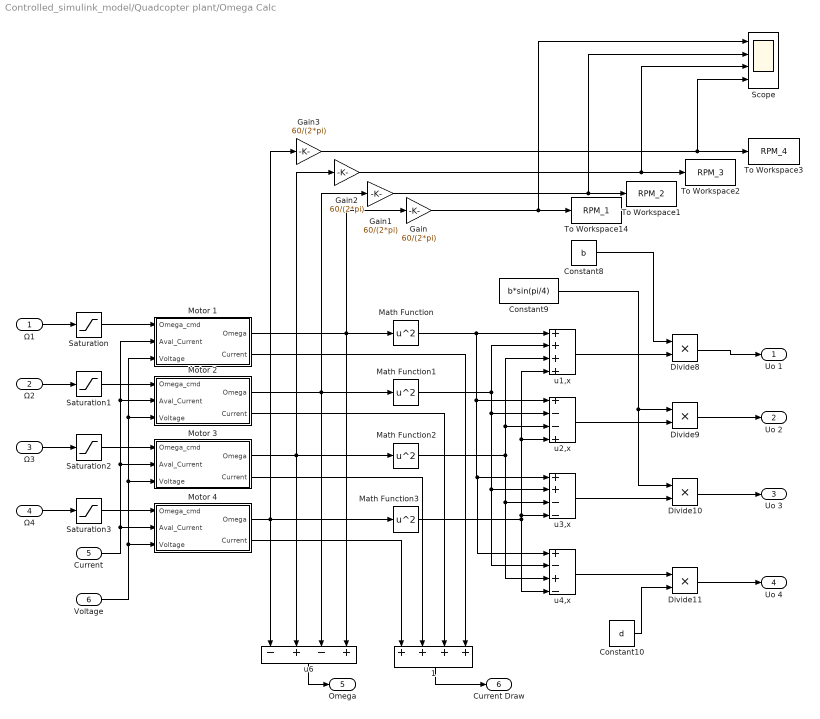
== system Controlled_simulink_model/Quadcopter plant/Omega Calc ==
  Ω1 : Inport
  Ω2 : Inport  Port=2
  Ω3 : Inport  Port=3
  Ω4 : Inport  Port=4
  Current : Inport  Port=5
  Voltage : Inport  Port=6
  " 1" : Sum  Inputs=++++
  " Motor 1" : Subsystem
  " Motor 2" : Subsystem
  " Motor 3" : Subsystem
  " Motor 4" : Subsystem
  Constant10 : Constant  Value=d
  Constant8 : Constant  Value=b
  Constant9 : Constant  Value=b*sin(pi/4)
  Divide{8..11} (4 alike) : Product  Inputs=**
  Gain{,1..3} (4 alike) : Gain  Gain=60/(2*pi)
  Math Function{,1..3} (4 alike) : Math  Operator=square  SignedPower=on  SaturateOnIntegerOverflow=on
  Saturation{,1..3} (4 alike) : Saturate  UpperLimit=inf  LowerLimit=0
  Scope : Scope  NumInputPorts=4
  To Workspace1 : ToWorkspace  VariableName=RPM_2  SampleTime=0.001
      settings: Save2DSignal=2-D array (concatenate along first dimension)
  To Workspace14 : ToWorkspace  VariableName=RPM_1  SampleTime=0.001
      settings: Save2DSignal=2-D array (concatenate along first dimension)
  To Workspace2 : ToWorkspace  VariableName=RPM_3  SampleTime=0.001
      settings: Save2DSignal=2-D array (concatenate along first dimension)
  To Workspace3 : ToWorkspace  VariableName=RPM_4  SampleTime=0.001
      settings: Save2DSignal=2-D array (concatenate along first dimension)
  u1,x : Sum  Inputs=++++
  u2,x : Sum  Inputs=+--+
  u3,x : Sum  Inputs=++--
  u4,x : Sum  Inputs=+-+-
  u6 : Sum  Inputs=-+-+
  Uo 1 : Outport  VectorParamsAs1DForOutWhenUnconnected=off
  Uo 2 : Outport  Port=2  VectorParamsAs1DForOutWhenUnconnected=off
  Uo 3 : Outport  Port=3  VectorParamsAs1DForOutWhenUnconnected=off
  Uo 4 : Outport  Port=4  VectorParamsAs1DForOutWhenUnconnected=off
  Omega : Outport  Port=5  VectorParamsAs1DForOutWhenUnconnected=off
  Current Draw : Outport  Port=6  VectorParamsAs1DForOutWhenUnconnected=off
  wires:
  Constant10/1 -> Divide11/2
  u4,x/1 -> Divide11/1
  u3,x/1 -> Divide10/2
  u2,x/1 -> Divide9/2
  Constant9/1 -> Divide10/1, Divide9/1
  u1,x/1 -> Divide8/2
  Constant8/1 -> Divide8/1
  u6/1 -> Omega/1
  Divide8/1 -> Uo 1/1
  Divide9/1 -> Uo 2/1
  Divide10/1 -> Uo 3/1
  Divide11/1 -> Uo 4/1
  " Motor 1"/1(Omega) -> Gain/1, u6/4, Math Function/1
  " Motor 2"/1(Omega) -> Gain1/1, u6/3, Math Function1/1
  " Motor 3"/1(Omega) -> Math Function2/1, Gain2/1, u6/2
  " Motor 4"/1(Omega) -> Math Function3/1, Gain3/1, u6/1
  " 1"/1 -> Current Draw/1
  Ω1/1 -> Saturation/1
  Ω2/1 -> Saturation1/1
  Ω3/1 -> Saturation2/1
  Ω4/1 -> Saturation3/1
  Saturation/1 -> " Motor 1"/1(Omega_cmd)
  Saturation1/1 -> " Motor 2"/1(Omega_cmd)
  Saturation2/1 -> " Motor 3"/1(Omega_cmd)
  Saturation3/1 -> " Motor 4"/1(Omega_cmd)
  Current/1 -> " Motor 4"/2(Aval_Current), " Motor 3"/2(Aval_Current), " Motor 2"/2(Aval_Current), " Motor 1"/2(Aval_Current)
  Voltage/1 -> " Motor 4"/3(Voltage), " Motor 3"/3(Voltage), " Motor 2"/3(Voltage), " Motor 1"/3(Voltage)
  " Motor 4"/2("Current ") -> " 1"/1
  " Motor 3"/2("Current ") -> " 1"/2
  " Motor 2"/2("Current ") -> " 1"/3
  " Motor 1"/2("Current ") -> " 1"/4
  Math Function/1 -> u4,x/1, u3,x/1, u2,x/1, u1,x/1
  Math Function1/1 -> u4,x/2, u3,x/2, u2,x/2, u1,x/2
  Math Function2/1 -> u4,x/3, u3,x/3, u1,x/3, u2,x/3
  Math Function3/1 -> u4,x/4, u1,x/4, u2,x/4, u3,x/4
  Gain/1 -> Scope/1, To Workspace14/1
  Gain1/1 -> Scope/2, To Workspace1/1
  Gain2/1 -> Scope/3, To Workspace2/1
  Gain3/1 -> Scope/4, To Workspace3/1

== system Controlled_simulink_model/Quadcopter plant/Angles->accels/Subsystem ==
  X_dot : Inport
  Phi : Inport  Port=2
  Theta : Inport  Port=3
  Psi : Inport  Port=4
  U1/M : Inport  Port=5
  Add : Sum  Inputs=+-
  Add1 : Sum  Inputs=+-
  Constant : Constant  Value=Ax/m
  Cos : Trigonometry  Operator=cos
  Cos1 : Trigonometry  Operator=cos
  Product : Product
  Product1 : Product  Inputs=3
  Product2 : Product
  Product3 : Product
  Sin : Trigonometry
  Sin1 : Trigonometry
  Sin2 : Trigonometry
  X_dot_dot : Outport  VectorParamsAs1DForOutWhenUnconnected=off
  wires:
  Product1/1 -> Add/2
  Product/1 -> Add/1
  U1/M/1 -> Product2/1
  Add/1 -> Product2/2
  Psi/1 -> Cos/1, Sin/1
  Phi/1 -> Cos1/1, Sin1/1
  Theta/1 -> Sin2/1
  Cos1/1 -> Product1/1
  Cos/1 -> Product1/2
  Sin2/1 -> Product1/3
  Sin1/1 -> Product/1
  Sin/1 -> Product/2
  Product2/1 -> Add1/1
  Add1/1 -> X_dot_dot/1
  X_dot/1 -> Product3/1
  Constant/1 -> Product3/2
  Product3/1 -> Add1/2

== system Controlled_simulink_model/Quadcopter plant/Angles->accels/Subsystem1 ==
  Y_dot : Inport
  Phi : Inport  Port=2
  Theta : Inport  Port=3
  Psi : Inport  Port=4
  U1/M : Inport  Port=5
  Add1 : Sum
  Add2 : Sum  Inputs=+-
  Constant : Constant  Value=Ay/m
  Cos : Trigonometry  Operator=cos
  Cos1 : Trigonometry  Operator=cos
  Product1 : Product
  Product3 : Product
  Product4 : Product  Inputs=3
  Product5 : Product
  Sin : Trigonometry
  Sin1 : Trigonometry
  Sin2 : Trigonometry
  Y_dot_dot : Outport  VectorParamsAs1DForOutWhenUnconnected=off
  wires:
  Psi/1 -> Sin/1, Cos/1
  Phi/1 -> Cos1/1, Sin1/1
  Theta/1 -> Sin2/1
  Add1/1 -> Product5/2
  Product4/1 -> Add1/2
  U1/M/1 -> Product5/1
  Product3/1 -> Add1/1
  Cos1/1 -> Product4/1
  Sin/1 -> Product4/2
  Sin2/1 -> Product4/3
  Sin1/1 -> Product3/1
  Cos/1 -> Product3/2
  Y_dot/1 -> Product1/1
  Constant/1 -> Product1/2
  Product1/1 -> Add2/2
  Product5/1 -> Add2/1
  Add2/1 -> Y_dot_dot/1

== system Controlled_simulink_model/Quadcopter plant/Angles->accels/Subsystem2 ==
  Z_dot : Inport
  Phi : Inport  Port=2
  Theta : Inport  Port=3
  U1/m : Inport  Port=4
  Add1 : Sum  Inputs=+-
  Add2 : Sum  Inputs=+-
  Constant : Constant  Value=Ay/m
  Constant2 : Constant  Value=g
  Cos : Trigonometry  Operator=cos
  Cos1 : Trigonometry  Operator=cos
  Product1 : Product
  Product6 : Product  Inputs=3
  Z_dot_dot : Outport  VectorParamsAs1DForOutWhenUnconnected=off
  wires:
  Phi/1 -> Cos1/1
  Theta/1 -> Cos/1
  U1/m/1 -> Product6/3
  Constant2/1 -> Add2/1
  Cos/1 -> Product6/1
  Product6/1 -> Add2/2
  Cos1/1 -> Product6/2
  Product1/1 -> Add1/2
  Z_dot/1 -> Product1/1
  Constant/1 -> Product1/2
  Add2/1 -> Add1/1
  Add1/1 -> Z_dot_dot/1

== system Controlled_simulink_model/Quadcopter plant/Inputs->ang_accel1/Subsystem ==
  U2 : Inport
  Theta_dot : Inport  Port=2
  Psi_dot : Inport  Port=3
  Ωr : Inport  Port=4
  Add : Sum  Inputs=+++
  Constant : Constant  Value=Iyy-Izz
  Constant1 : Constant  Value=Jr
  Constant2 : Constant  Value=l
  Constant3 : Constant  Value=Ixx
  Divide : Product  Inputs=*/
  Product : Product  Inputs=3
  Product1 : Product  Inputs=3
  Product2 : Product
  Phi_dot_dot : Outport  VectorParamsAs1DForOutWhenUnconnected=off
  wires:
  Psi_dot/1 -> Product/2
  Theta_dot/1 -> Product/1, Product1/3
  Constant/1 -> Product/3
  Ωr/1 -> Product1/2
  Constant1/1 -> Product1/1
  U2/1 -> Product2/2
  Constant2/1 -> Product2/1
  Product1/1 -> Add/2
  Product2/1 -> Add/1
  Product/1 -> Add/3
  Add/1 -> Divide/1
  Constant3/1 -> Divide/2
  Divide/1 -> Phi_dot_dot/1

== system Controlled_simulink_model/Quadcopter plant/Inputs->ang_accel1/Subsystem1 ==
  Phi_dot : Inport
  Theta_dot : Inport  Port=2
  U4 : Inport  Port=3
  Add2 : Sum
  Constant11 : Constant  Value=Izz
  Constant8 : Constant  Value=Ixx-Iyy
  Divide2 : Product  Inputs=*/
  Product6 : Product  Inputs=3
  Psi_dot_dot : Outport  VectorParamsAs1DForOutWhenUnconnected=off
  wires:
  Theta_dot/1 -> Product6/1
  Phi_dot/1 -> Product6/2
  Constant8/1 -> Product6/3
  Add2/1 -> Divide2/1
  Constant11/1 -> Divide2/2
  Divide2/1 -> Psi_dot_dot/1
  Product6/1 -> Add2/2
  U4/1 -> Add2/1

== system Controlled_simulink_model/Quadcopter plant/Inputs->ang_accel1/Subsystem2 ==
  Ωr : Inport
  Psi_dot : Inport  Port=2
  U3 : Inport  Port=3
  Phi_dot : Inport  Port=4
  Add1 : Sum  Inputs=+-+
  Constant4 : Constant  Value=Izz-Ixx
  Constant5 : Constant  Value=Jr
  Constant6 : Constant  Value=l
  Constant7 : Constant  Value=Iyy
  Divide1 : Product  Inputs=*/
  Product3 : Product  Inputs=3
  Product4 : Product  Inputs=3
  Product5 : Product
  Theta_dot_dot : Outport  VectorParamsAs1DForOutWhenUnconnected=off
  wires:
  Psi_dot/1 -> Product3/2
  Phi_dot/1 -> Product4/3, Product3/1
  Ωr/1 -> Product4/2
  Constant4/1 -> Product3/3
  Constant5/1 -> Product4/1
  U3/1 -> Product5/2
  Constant6/1 -> Product5/1
  Product4/1 -> Add1/2
  Product5/1 -> Add1/1
  Product3/1 -> Add1/3
  Add1/1 -> Divide1/1
  Constant7/1 -> Divide1/2
  Divide1/1 -> Theta_dot_dot/1

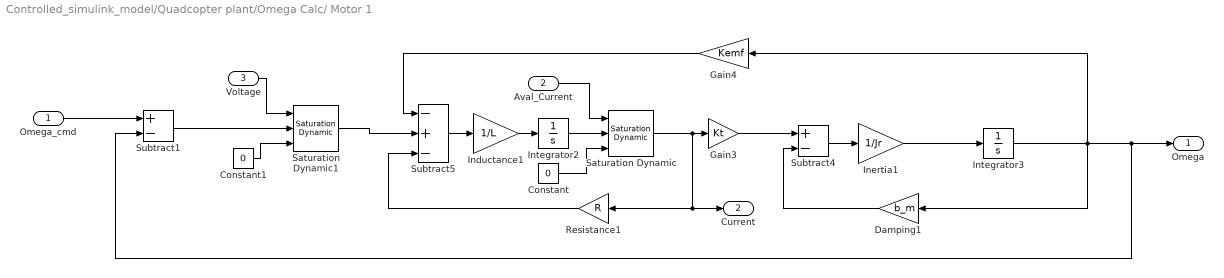
== system Controlled_simulink_model/Quadcopter plant/Omega Calc/ Motor 1 ==
  Omega_cmd : Inport
  Aval_Current : Inport  Port=2
  Voltage : Inport  Port=3
  Constant : Constant  Value=0
  Constant1 : Constant  Value=0
  Damping1 : Gain  Gain=b_m
  Gain3 : Gain  Gain=Kt
  Gain4 : Gain  Gain=Kemf
  Inductance1 : Gain  Gain=1/L
  Inertia1 : Gain  Gain=1/Jr
  Integrator2 : Integrator  LimitOutput=on  LowerSaturationLimit=0
  Integrator3 : Integrator  LimitOutput=on  LowerSaturationLimit=0
  Resistance1 : Gain  Gain=R
  Saturation Dynamic : simulink/Discontinuities/Saturation Dynamic  OutMin=[]  OutMax=[]  OutDataTypeStr=Inherit: Same as second input  OutDataType=fixdt(1, 16)  OutScaling=2^-10  DoSatur=off
  Saturation Dynamic1 : simulink/Discontinuities/Saturation Dynamic  OutMin=[]  OutMax=[]  OutDataTypeStr=Inherit: Same as second input  OutDataType=fixdt(1, 16)  OutScaling=2^-10  DoSatur=off
  Subtract1 : Sum  Inputs=+-
  Subtract4 : Sum  Inputs=+-
  Subtract5 : Sum  Inputs=-+-
  Omega : Outport  VectorParamsAs1DForOutWhenUnconnected=off
  "Current " : Outport  Port=2  VectorParamsAs1DForOutWhenUnconnected=off
  wires:
  Inductance1/1 -> Integrator2/1
  Inertia1/1 -> Integrator3/1
  Resistance1/1 -> Subtract5/3
  Damping1/1 -> Subtract4/2
  Subtract5/1 -> Inductance1/1
  Saturation Dynamic1/1 -> Subtract5/2
  Gain4/1 -> Subtract5/1
  Subtract4/1 -> Inertia1/1
  Gain3/1 -> Subtract4/1
  Omega_cmd/1 -> Subtract1/1
  Integrator3/1 -> Subtract1/2, Omega/1, Damping1/1, Gain4/1
  Constant/1 -> Saturation Dynamic/3
  Aval_Current/1 -> Saturation Dynamic/1
  Integrator2/1 -> Saturation Dynamic/2
  Voltage/1 -> Saturation Dynamic1/1
  Constant1/1 -> Saturation Dynamic1/3
  Subtract1/1 -> Saturation Dynamic1/2
  Saturation Dynamic/1 -> Resistance1/1, "Current "/1, Gain3/1

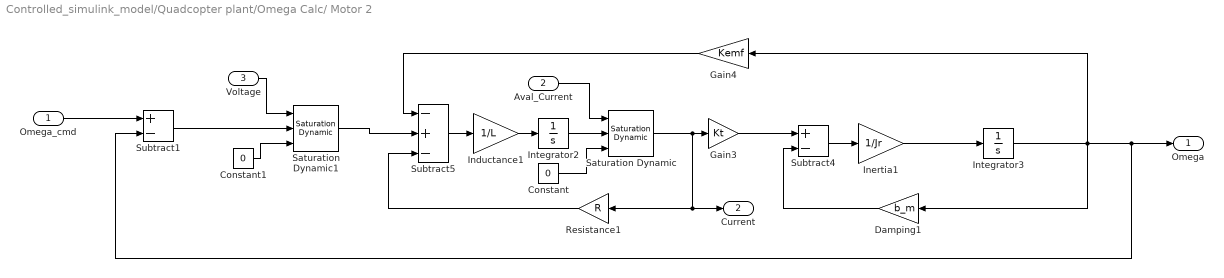
== system Controlled_simulink_model/Quadcopter plant/Omega Calc/ Motor 2 ==
  Omega_cmd : Inport
  Aval_Current : Inport  Port=2
  Voltage : Inport  Port=3
  Constant : Constant  Value=0
  Constant1 : Constant  Value=0
  Damping1 : Gain  Gain=b_m
  Gain3 : Gain  Gain=Kt
  Gain4 : Gain  Gain=Kemf
  Inductance1 : Gain  Gain=1/L
  Inertia1 : Gain  Gain=1/Jr
  Integrator2 : Integrator  LimitOutput=on  LowerSaturationLimit=0
  Integrator3 : Integrator  LimitOutput=on  LowerSaturationLimit=0
  Resistance1 : Gain  Gain=R
  Saturation Dynamic : simulink/Discontinuities/Saturation Dynamic  OutMin=[]  OutMax=[]  OutDataTypeStr=Inherit: Same as second input  OutDataType=fixdt(1, 16)  OutScaling=2^-10  DoSatur=off
  Saturation Dynamic1 : simulink/Discontinuities/Saturation Dynamic  OutMin=[]  OutMax=[]  OutDataTypeStr=Inherit: Same as second input  OutDataType=fixdt(1, 16)  OutScaling=2^-10  DoSatur=off
  Subtract1 : Sum  Inputs=+-
  Subtract4 : Sum  Inputs=+-
  Subtract5 : Sum  Inputs=-+-
  Omega : Outport  VectorParamsAs1DForOutWhenUnconnected=off
  "Current " : Outport  Port=2  VectorParamsAs1DForOutWhenUnconnected=off
  wires:
  Inductance1/1 -> Integrator2/1
  Inertia1/1 -> Integrator3/1
  Resistance1/1 -> Subtract5/3
  Damping1/1 -> Subtract4/2
  Subtract5/1 -> Inductance1/1
  Saturation Dynamic1/1 -> Subtract5/2
  Gain4/1 -> Subtract5/1
  Subtract4/1 -> Inertia1/1
  Gain3/1 -> Subtract4/1
  Omega_cmd/1 -> Subtract1/1
  Integrator3/1 -> Subtract1/2, Omega/1, Damping1/1, Gain4/1
  Constant/1 -> Saturation Dynamic/3
  Aval_Current/1 -> Saturation Dynamic/1
  Integrator2/1 -> Saturation Dynamic/2
  Voltage/1 -> Saturation Dynamic1/1
  Constant1/1 -> Saturation Dynamic1/3
  Subtract1/1 -> Saturation Dynamic1/2
  Saturation Dynamic/1 -> Resistance1/1, "Current "/1, Gain3/1

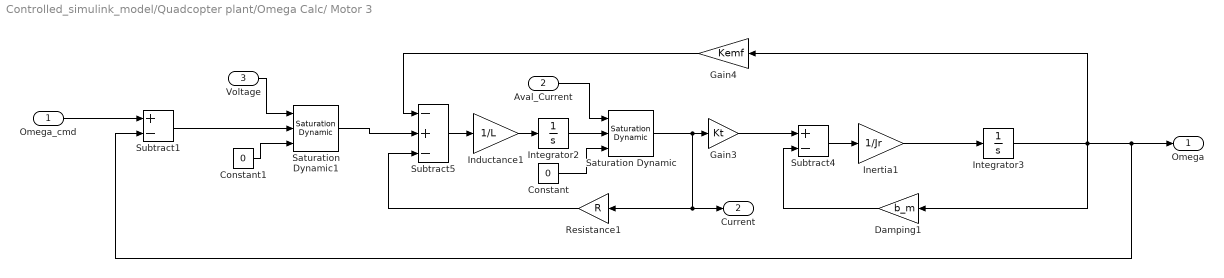
== system Controlled_simulink_model/Quadcopter plant/Omega Calc/ Motor 3 ==
  Omega_cmd : Inport
  Aval_Current : Inport  Port=2
  Voltage : Inport  Port=3
  Constant : Constant  Value=0
  Constant1 : Constant  Value=0
  Damping1 : Gain  Gain=b_m
  Gain3 : Gain  Gain=Kt
  Gain4 : Gain  Gain=Kemf
  Inductance1 : Gain  Gain=1/L
  Inertia1 : Gain  Gain=1/Jr
  Integrator2 : Integrator  LimitOutput=on  LowerSaturationLimit=0
  Integrator3 : Integrator  LimitOutput=on  LowerSaturationLimit=0
  Resistance1 : Gain  Gain=R
  Saturation Dynamic : simulink/Discontinuities/Saturation Dynamic  OutMin=[]  OutMax=[]  OutDataTypeStr=Inherit: Same as second input  OutDataType=fixdt(1, 16)  OutScaling=2^-10  DoSatur=off
  Saturation Dynamic1 : simulink/Discontinuities/Saturation Dynamic  OutMin=[]  OutMax=[]  OutDataTypeStr=Inherit: Same as second input  OutDataType=fixdt(1, 16)  OutScaling=2^-10  DoSatur=off
  Subtract1 : Sum  Inputs=+-
  Subtract4 : Sum  Inputs=+-
  Subtract5 : Sum  Inputs=-+-
  Omega : Outport  VectorParamsAs1DForOutWhenUnconnected=off
  "Current " : Outport  Port=2  VectorParamsAs1DForOutWhenUnconnected=off
  wires:
  Inductance1/1 -> Integrator2/1
  Inertia1/1 -> Integrator3/1
  Resistance1/1 -> Subtract5/3
  Damping1/1 -> Subtract4/2
  Subtract5/1 -> Inductance1/1
  Saturation Dynamic1/1 -> Subtract5/2
  Gain4/1 -> Subtract5/1
  Subtract4/1 -> Inertia1/1
  Gain3/1 -> Subtract4/1
  Omega_cmd/1 -> Subtract1/1
  Integrator3/1 -> Subtract1/2, Omega/1, Damping1/1, Gain4/1
  Constant/1 -> Saturation Dynamic/3
  Aval_Current/1 -> Saturation Dynamic/1
  Integrator2/1 -> Saturation Dynamic/2
  Voltage/1 -> Saturation Dynamic1/1
  Constant1/1 -> Saturation Dynamic1/3
  Subtract1/1 -> Saturation Dynamic1/2
  Saturation Dynamic/1 -> Resistance1/1, "Current "/1, Gain3/1

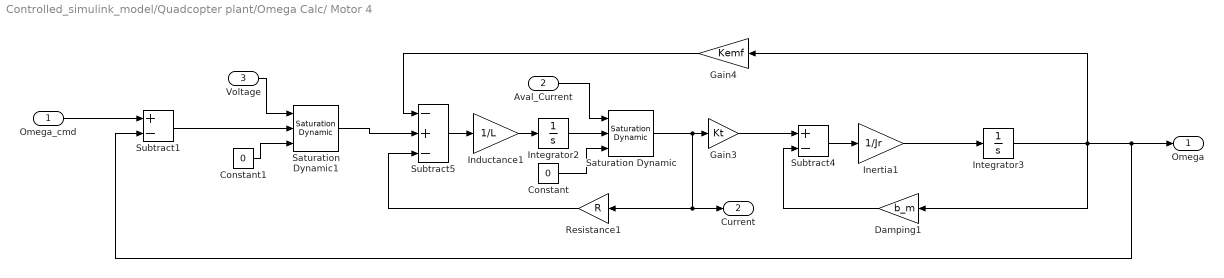
== system Controlled_simulink_model/Quadcopter plant/Omega Calc/ Motor 4 ==
  Omega_cmd : Inport
  Aval_Current : Inport  Port=2
  Voltage : Inport  Port=3
  Constant : Constant  Value=0
  Constant1 : Constant  Value=0
  Damping1 : Gain  Gain=b_m
  Gain3 : Gain  Gain=Kt
  Gain4 : Gain  Gain=Kemf
  Inductance1 : Gain  Gain=1/L
  Inertia1 : Gain  Gain=1/Jr
  Integrator2 : Integrator  LimitOutput=on  LowerSaturationLimit=0
  Integrator3 : Integrator  LimitOutput=on  LowerSaturationLimit=0
  Resistance1 : Gain  Gain=R
  Saturation Dynamic : simulink/Discontinuities/Saturation Dynamic  OutMin=[]  OutMax=[]  OutDataTypeStr=Inherit: Same as second input  OutDataType=fixdt(1, 16)  OutScaling=2^-10  DoSatur=off
  Saturation Dynamic1 : simulink/Discontinuities/Saturation Dynamic  OutMin=[]  OutMax=[]  OutDataTypeStr=Inherit: Same as second input  OutDataType=fixdt(1, 16)  OutScaling=2^-10  DoSatur=off
  Subtract1 : Sum  Inputs=+-
  Subtract4 : Sum  Inputs=+-
  Subtract5 : Sum  Inputs=-+-
  Omega : Outport  VectorParamsAs1DForOutWhenUnconnected=off
  "Current " : Outport  Port=2  VectorParamsAs1DForOutWhenUnconnected=off
  wires:
  Inductance1/1 -> Integrator2/1
  Inertia1/1 -> Integrator3/1
  Resistance1/1 -> Subtract5/3
  Damping1/1 -> Subtract4/2
  Subtract5/1 -> Inductance1/1
  Saturation Dynamic1/1 -> Subtract5/2
  Gain4/1 -> Subtract5/1
  Subtract4/1 -> Inertia1/1
  Gain3/1 -> Subtract4/1
  Omega_cmd/1 -> Subtract1/1
  Integrator3/1 -> Subtract1/2, Omega/1, Damping1/1, Gain4/1
  Constant/1 -> Saturation Dynamic/3
  Aval_Current/1 -> Saturation Dynamic/1
  Integrator2/1 -> Saturation Dynamic/2
  Voltage/1 -> Saturation Dynamic1/1
  Constant1/1 -> Saturation Dynamic1/3
  Subtract1/1 -> Saturation Dynamic1/2
  Saturation Dynamic/1 -> Resistance1/1, "Current "/1, Gain3/1

== matlab function Controlled_simulink_model/IMU/MATLAB Function ==
  data: Xdd input; Ydd input; Zdd input; Phi input; Accel_vec output; Theta input; Psi input
function Accel_vec = World2Body(Xdd,Ydd,Zdd,Phi,Theta,Psi)

Trans_mat=[(cos(Psi)*cos(Theta)), (-sin(Psi)*cos(Phi)+cos(Psi)*sin(Theta)*sin(Phi)), (sin(Psi)*sin(Phi)+cos(Psi)*sin(Theta)*cos(Phi));...
          (sin(Psi)*cos(Theta)), (cos(Psi)*cos(Phi)+sin(Theta)*sin(Psi)*sin(Phi)), (-cos(Psi)*sin(Phi)+sin(Theta)*sin(Psi)*cos(Phi));...
          (-sin(Theta)), (cos(Theta)*sin(Phi)), (cos(Theta)*cos(Phi))];
      
Accel_world=[Xdd;Ydd;Zdd];
Accel_vec=(Trans_mat^-1)*Accel_world;
